simulink model "aufgabe_b3"  (R2016b)
settings: Solver=VariableStepAuto  StartTime=0.0  StopTime=10.0  RelTol=1e-3
settings Model: Creator=Thomas  LastModifiedBy=Thomas

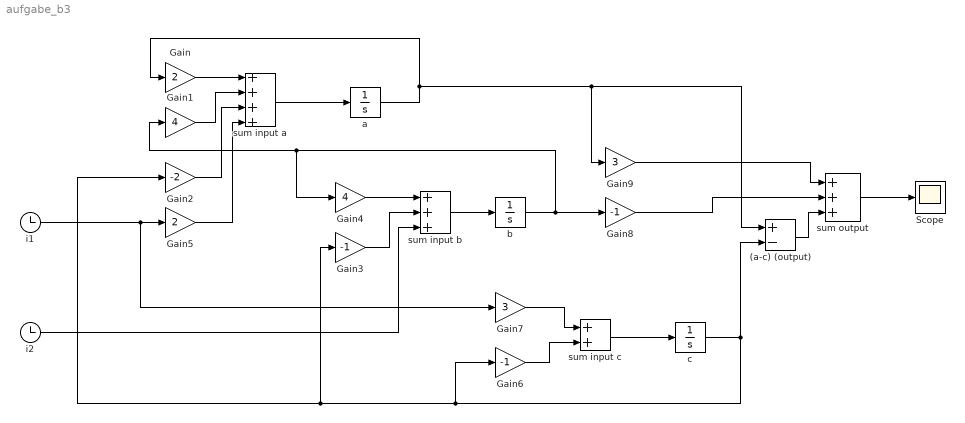
== system aufgabe_b3 ==
  (a-c) (output) : Sum  Inputs=+-
  Gain : Gain  Gain=2
  Gain1 : Gain  Gain=4
  Gain2 : Gain  Gain=-2
  Gain3 : Gain  Gain=-1
  Gain4 : Gain  Gain=4
  Gain5 : Gain  Gain=2
  Gain6 : Gain  Gain=-1
  Gain7 : Gain  Gain=3
  Gain8 : Gain  Gain=-1
  Gain9 : Gain  Gain=3
  Scope : Scope
  a : Integrator
  b : Integrator
  c : Integrator
  i1 : Clock
  i2 : Clock
  sum input a : Sum  Inputs=++++
  sum input b : Sum  Inputs=+++
  sum input c : Sum
  sum output : Sum  Inputs=+++
  wires:
  sum input a/1 -> a/1
  a/1 -> Gain/1, (a-c) (output)/1, Gain9/1
  sum input b/1 -> b/1
  b/1 -> Gain8/1, Gain4/1, Gain1/1
  sum input c/1 -> c/1
  c/1 -> Gain3/1, Gain2/1, Gain6/1, (a-c) (output)/2
  i1/1 -> Gain7/1, Gain5/1
  i2/1 -> sum input b/3
  sum output/1 -> Scope/1
  (a-c) (output)/1 -> sum output/3
  Gain/1 -> sum input a/1
  Gain1/1 -> sum input a/2
  Gain2/1 -> sum input a/3
  Gain5/1 -> sum input a/4
  Gain4/1 -> sum input b/1
  Gain3/1 -> sum input b/2
  Gain7/1 -> sum input c/1
  Gain6/1 -> sum input c/2
  Gain9/1 -> sum output/1
  Gain8/1 -> sum output/2
